simulink model "Copy_of_mVeh_fun_tbm"  (R2020a)
settings: configuration reference "config_10ms" (kept outside this file)
undefined symbols (not defined in the file): Calib_tbmVeh_drCmdMcP_incRate, Calib_tbmVeh_drCmdMcP_tgt, Calib_tbmVeh_set1_x4, Calib_tbmVeh_set2_x4, Parm_tbmVeh_sig_max_numInvalid, Parm_tbmVeh_sig_tolerate_numInvalid
libraries: canmsglib x7, speedgoatlib_IO691 x6, simulink x2, lib_signals_to_nByteLayout_withCrc x2, lib_cal_CAN_msgCount x2
settings Model: PauseTimes=49.73  NumberOfSteps=20  Creator=jianjun.gao  LastModifiedBy=bowen.zheng
settings ConfigSetRef: SourceName=config_10ms  SourceLocation=Base Workspace

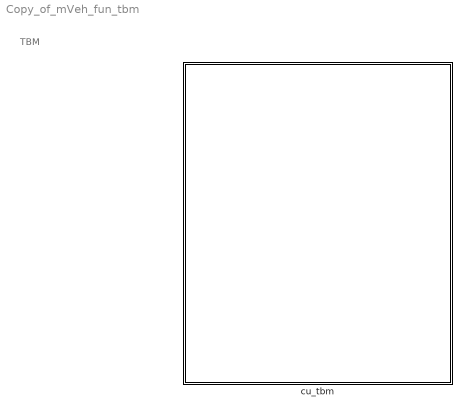
== system Copy_of_mVeh_fun_tbm ==
  note: TBM
  cu_tbm : Subsystem

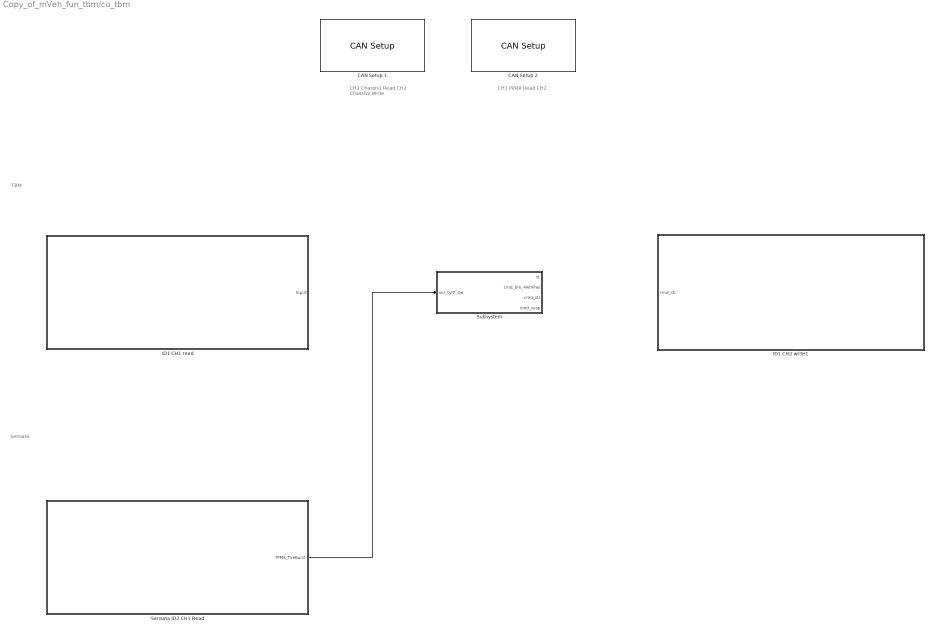
== system Copy_of_mVeh_fun_tbm/cu_tbm ==
  note: CH1 PVRR Read
      | CH2
  note: CH1 Chassis1 Read
      | CH2 Chassis2 Write
  note: Sensata
  note: TBM
  CAN Setup 1 : speedgoatlib_IO691/CAN Setup   moduletype=IO691  id=1  pciSlot=[12 0]  chn1=CAN (HS)  chn2=CAN (HS)  chn3=Disabled  chn4=Disabled  initStruct=[]  termStruct=[]  ArbitrationbdrChn1=500 kBaud  ArbitrationManbdrChn1=[2,16,63,16]  FdbdrChn1=5.0 MBaud  FdManbdrChn1=[2,2,5,2]  ArbitrationbdrChn2=500 kBaud  ArbitrationManbdrChn2=[2,16,63,16]  FdbdrChn2=5.0 MBaud  FdManbdrChn2=[2,2,5,2]  ArbitrationbdrChn3=1.0 MBaud  ArbitrationManbdrChn3=[2,8,31,8]  FdbdrChn3=5.0 MBaud  FdManbdrChn3=[2,2,5,2]  ArbitrationbdrChn4=1.0 MBaud  ArbitrationManbdrChn4=[2,8,31,8]  FdbdrChn4=5.0 MBaud  FdManbdrChn4=[2,2,5,2]  moduleInitValues=[691 1 12 0]
      settings: SourceProductName=Simulink Real-Time: Speedgoat I/O Blockset
  CAN Setup 2 : speedgoatlib_IO691/CAN Setup   moduletype=IO691  id=2  pciSlot=[7 0]  chn1=CAN (HS)  chn2=CAN (HS)  chn3=Disabled  chn4=Disabled  initStruct=[]  termStruct=[]  ArbitrationbdrChn1=500 kBaud  ArbitrationManbdrChn1=[2,16,63,16]  FdbdrChn1=5.0 MBaud  FdManbdrChn1=[2,2,5,2]  ArbitrationbdrChn2=500 kBaud  ArbitrationManbdrChn2=[2,16,63,16]  FdbdrChn2=5.0 MBaud  FdManbdrChn2=[2,2,5,2]  ArbitrationbdrChn3=1.0 MBaud  ArbitrationManbdrChn3=[2,8,31,8]  FdbdrChn3=5.0 MBaud  FdManbdrChn3=[2,2,5,2]  ArbitrationbdrChn4=1.0 MBaud  ArbitrationManbdrChn4=[2,8,31,8]  FdbdrChn4=5.0 MBaud  FdManbdrChn4=[2,2,5,2]  moduleInitValues=[691 2 7 0]
      settings: SourceProductName=Simulink Real-Time: Speedgoat I/O Blockset
  ID1 CH1 read : Subsystem
  ID1 CH2 write1 : Subsystem
  Sensata ID2 CH1 Read : Subsystem
  Subsystem : Subsystem
  wires:
  Sensata ID2 CH1 Read/1(TPMS_TireBurst) -> Subsystem/1(snr_tyrP_4w)

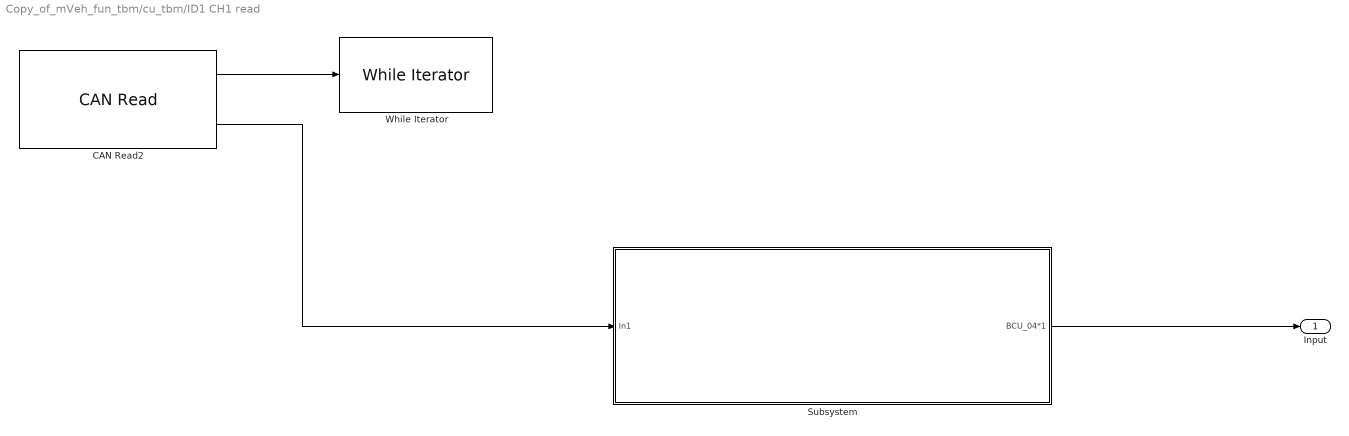
== system Copy_of_mVeh_fun_tbm/cu_tbm/ID1 CH1 read ==
  CAN Read2 : speedgoatlib_IO691/CAN Read  id=1  ts=-1  channel=1  messageType=CAN  canType=CAN (HS)  initValues=[691 1 -1 0 1 1]
      settings: SourceProductName=Simulink Real-Time: Speedgoat I/O Blockset
  Subsystem : Subsystem
  While Iterator : WhileIterator  MaxIters=-1  WhileBlockType=do-while
  Input : Outport
  wires:
  CAN Read2/1 -> While Iterator/1
  CAN Read2/2 -> Subsystem/1(In1)
  Subsystem/1(BCU_04*1) -> Input/1

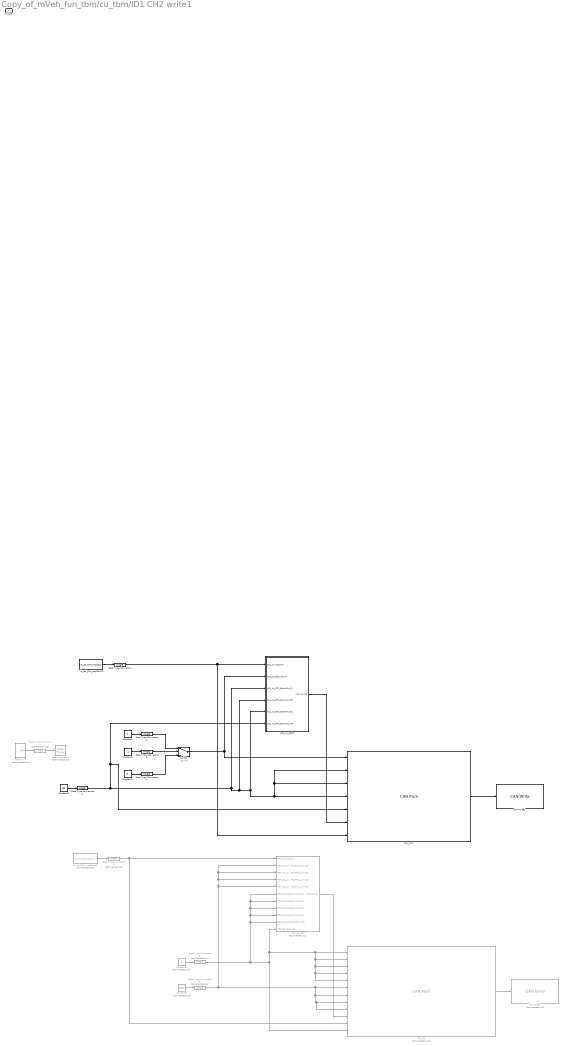
== system Copy_of_mVeh_fun_tbm/cu_tbm/ID1 CH2 write1 ==
  cmd_str : Inport
  CAN Write1 : speedgoatlib_IO691/CAN Write  id=1  ts=0.01  channel=2  messageType=CAN  enableStatusPort=off  canType=CAN (HS)  initValues=[691 1 0.01 1 1 1 0]
      settings: SourceProductName=Simulink Real-Time: Speedgoat I/O Blockset
  CAN Write2 : speedgoatlib_IO691/CAN Write  Commented=on  id=1  ts=0.01  channel=2  messageType=CAN  enableStatusPort=off  canType=CAN (HS)  initValues=[691 1 0.01 1 1 1 0]
      settings: SourceProductName=Simulink Real-Time: Speedgoat I/O Blockset
  Constant : Constant
  Constant1 : Constant  Value=0
  Constant2 : Constant  Value=80
  Constant3 : Constant  Commented=on  Value=2000
  Constant4 : Constant  Value=-1
  Constant6 : Constant  Commented=on
  Data Type Conversion{,2,4,7..8} (5 alike) : DataTypeConversion  OutDataTypeStr=single
  Data Type Conversion{1,3,5..6} (4 alike) : DataTypeConversion  Commented=on  OutDataTypeStr=single
  Gain (t) : Subsystem  Commented=on
  Rate Transition2 : RateTransition  Commented=on
  Switch : Switch  Criteria=u2 > Threshold
  TBM_02 : canmsglib/CAN Pack  Commented=on  CANdbFile=D:\spdGoat_prj_20221209\mVeh_fun_tbm_20221209\support\dbc\FCC1_NT2_Chassis1_CAN_Official_Release_V_1_4_DA_01_updated_mod.dbc  MsgList=TBM_02  MsgName=TBM_02  MsgIDType=Standard (11-bit identifier)  MsgIdentifier=128  MsgLength=8  Remote=off  ApplyMinMax=off  BusOutput=off  SignalInfo={'LeakActv_spring1','56','1','BE','unsigned','Standard','0','1','0','0','1';'LeakActv_spring2','57','1','BE','unsigned','Standard','0','1','0','0','1';'LeakActv_spring3','58','1','BE','unsigned','Standard','0','1','0','0','1';'LeakActv_spring4','59','1','BE','unsigned','Standard','0','1','0','0','1';'LeakFirst_springID','60','3','BE','unsigned','Standard','0','1','0','0','7';'LeakTargPres_spring1','17','11','BE','unsigned','Standard','0','1','0','0','2047';'LeakTargPres_spring2','38','11','BE','unsigned','Standard','0','1','0','0','2047';'LeakTargPres_spring3','43','11','BE','unsigned','Standard','0','1','0','0','2047';'LeakTargPres_spring4','48','11','BE','unsigned','Standard','0','1','0','0','2047';'TBM_02_CRC','0','8','BE','unsigned','Standard','0','1','0','0','255';'TBM_02_MsgCntr','12','4','BE','unsigned','Standard','0','1','0','0','15';'TBM_02_reserved','63','1','BE','unsigned','Standard','0','1','0','0','1'}
      settings: SourceProductBaseCode=ME,VN  DataFormat=CANdb specified signals
  TBM_02_CRC : Subsystem  Commented=on
  VCU_14*1 : canmsglib/CAN Pack  CANdbFile=D:\spdGoat_prj_20221209\mVeh_fun_tbm_20221209\support\dbc\NIO_NT2_Chassis2_CAN_Official_Release_V_1_1_DA_02.dbc  MsgList=VCU_14  MsgName=VCU_14  MsgIDType=Standard (11-bit identifier)  MsgIdentifier=75  MsgLength=8  Remote=off  ApplyMinMax=off  BusOutput=off  SignalInfo={'BTS_Active','23','1','BE','unsigned','Standard','0','1','0','0','1';'BTS_BrakeTar_FL','16','7','BE','unsigned','Standard','0','1','0','0','127';'BTS_BrakeTar_FR','25','7','BE','unsigned','Standard','0','1','0','0','127';'BTS_BrakeTar_RL','34','7','BE','unsigned','Standard','0','1','0','0','127';'BTS_BrakeTar_RR','43','7','BE','unsigned','Standard','0','1','0','0','127';'VCU_14_CRC','0','8','BE','unsigned','Standard','0','1','0','0','255';'VCU_14_MsgCntr','12','4','BE','unsigned','Standard','0','1','0','0','15'}
      settings: SourceProductBaseCode=ME,VN  DataFormat=CANdb specified signals
  VCU_14_CRC1 : Subsystem
  lib_cal_CAN_msgCount : lib_cal_CAN_msgCount/lib_cal_CAN_msgCount  SystemSampleTime=-1  Latency=0  AutoFrameSizeCalculation=off
  lib_cal_CAN_msgCount1 : lib_cal_CAN_msgCount/lib_cal_CAN_msgCount  Commented=on  SystemSampleTime=-1  Latency=0  AutoFrameSizeCalculation=off
  wires:
  Gain (t)/1("Gain ") -> Data Type Conversion1/1
  Constant/1 -> Data Type Conversion4/1
  Constant1/1 -> Data Type Conversion7/1
  Switch/1 -> VCU_14*1/1, VCU_14_CRC1/2("VCU_14_BTS_Active ")
  Constant2/1 -> Data Type Conversion2/1
  VCU_14_CRC1/1(VCU_14_crc) -> VCU_14*1/6
  Data Type Conversion/1 -> VCU_14*1/7, VCU_14_CRC1/1("VCU_14_MsgCntr ")
  lib_cal_CAN_msgCount/1 -> Data Type Conversion/1
  VCU_14*1/1 -> CAN Write1/1
  Data Type Conversion1/1 -> Rate Transition2/1
  Data Type Conversion2/1 -> VCU_14_CRC1/6("VCU_14_BTS_BrakeTar_RR "), VCU_14*1/5, VCU_14_CRC1/4("VCU_14_BTS_BrakeTar_FR "), VCU_14_CRC1/5("VCU_14_BTS_BrakeTar_RL "), VCU_14*1/2, VCU_14*1/3, VCU_14*1/4, VCU_14_CRC1/3("VCU_14_BTS_BrakeTar_FL ")
  TBM_02/1 -> CAN Write2/1
  Constant6/1 -> Data Type Conversion5/1
  TBM_02_CRC/1(TBM_02_crc) -> TBM_02/10
  lib_cal_CAN_msgCount1/1 -> Data Type Conversion3/1
  Constant3/1 -> Data Type Conversion6/1
  Data Type Conversion6/1 -> TBM_02_CRC/5("TBM_02_LeakTargPres_spring4 "), TBM_02_CRC/4("TBM_02_LeakTargPres_spring3 "), TBM_02_CRC/3("TBM_02_LeakTargPres_spring1 "), TBM_02_CRC/2("TBM_02_LeakTargPres_spring2 "), TBM_02/9, TBM_02/8, TBM_02/7, TBM_02/6
  Data Type Conversion3/1 -> TBM_02/11, TBM_02_CRC/1("TBM_02_MsgCntr ")
  Data Type Conversion5/1 -> TBM_02_CRC/10(TBM_02_LeakFirst_springID), TBM_02_CRC/9(TBM_02_LeakActv_spring3), TBM_02_CRC/8("TBM_02_LeakActv_spring4 "), TBM_02_CRC/6(TBM_02_LeakActv_spring2), TBM_02_CRC/7("TBM_02_LeakActv_spring1 "), TBM_02/12, TBM_02_CRC/11(TBM_02_reserved), TBM_02/5, TBM_02/4, TBM_02/3, TBM_02/2, TBM_02/1
  Data Type Conversion4/1 -> Switch/1
  Data Type Conversion7/1 -> Switch/3
  Constant4/1 -> Data Type Conversion8/1
  Data Type Conversion8/1 -> Switch/2

== system Copy_of_mVeh_fun_tbm/cu_tbm/Sensata ID2 CH1 Read ==
  CAN Read2 : speedgoatlib_IO691/CAN Read  id=2  ts=-1  channel=1  messageType=CAN  canType=CAN (HS)  initValues=[691 2 -1 0 1 1]
      settings: SourceProductName=Simulink Real-Time: Speedgoat I/O Blockset
  Subsystem : Subsystem
  While Iterator : WhileIterator  MaxIters=-1  WhileBlockType=do-while
  TPMS_TireBurst : Outport
  wires:
  CAN Read2/1 -> While Iterator/1
  CAN Read2/2 -> Subsystem/1(In1)
  Subsystem/1(TPMS_TireBurst) -> TPMS_TireBurst/1

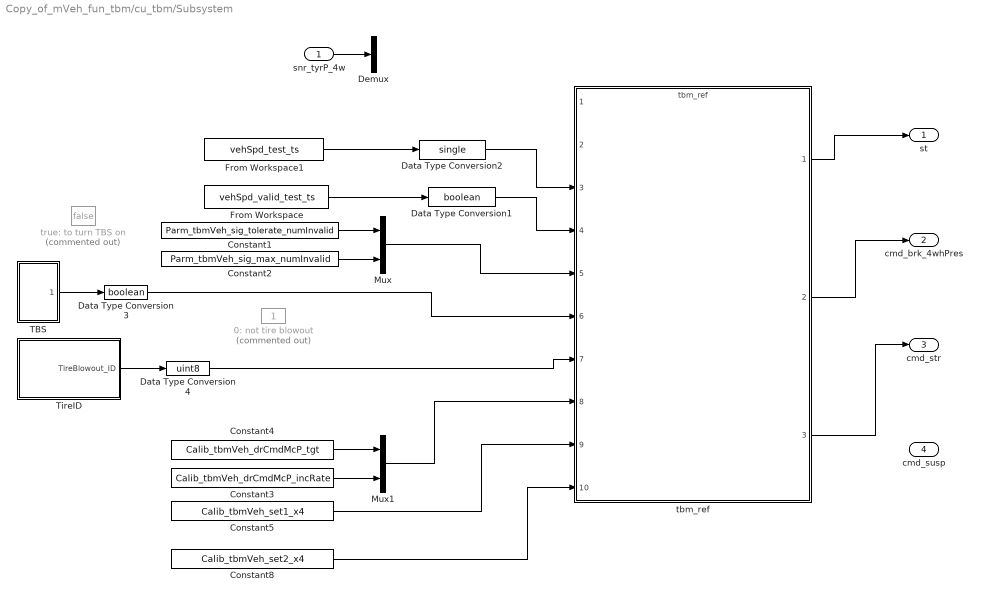
== system Copy_of_mVeh_fun_tbm/cu_tbm/Subsystem ==
  snr_tyrP_4w : Inport
  0: not tire blowout : Constant  Commented=on  OutDataTypeStr=uint8  SampleTime=-1
  Constant1 : Constant  Value=Parm_tbmVeh_sig_tolerate_numInvalid  OutDataTypeStr=int8  SampleTime=-1
  Constant2 : Constant  Value=Parm_tbmVeh_sig_max_numInvalid  OutDataTypeStr=int8  SampleTime=-1
  Constant3 : Constant  Value=Calib_tbmVeh_drCmdMcP_incRate  OutDataTypeStr=single  SampleTime=-1
  Constant4 : Constant  Value=Calib_tbmVeh_drCmdMcP_tgt  OutDataTypeStr=single  SampleTime=-1
  Constant5 : Constant  Value=Calib_tbmVeh_set1_x4  OutDataTypeStr=single  SampleTime=-1
  Constant8 : Constant  Value=Calib_tbmVeh_set2_x4  OutDataTypeStr=single  SampleTime=-1
  Data Type Conversion1 : DataTypeConversion  OutDataTypeStr=boolean
  Data Type Conversion2 : DataTypeConversion  OutDataTypeStr=single
  Data Type Conversion3 : DataTypeConversion  OutDataTypeStr=boolean
  Data Type Conversion4 : DataTypeConversion  OutDataTypeStr=uint8
  Demux : Demux  Outputs=2
  From Workspace : FromWorkspace  VariableName=vehSpd_valid_test_ts
  From Workspace1 : FromWorkspace  VariableName=vehSpd_test_ts
  Mux : Mux  Inputs=2
  Mux1 : Mux  Inputs=2
  TBS : Subsystem
  TireID : Subsystem
  tbm_ref : ModelReference  ModelNameDialog=tbm_ref.slx  SimulationMode=Normal  ModelReferenceVersion=1.657
  true: to turn TBS on : Constant  Commented=on  Value=false  OutDataTypeStr=boolean  SampleTime=-1
  st : Outport
  cmd_brk_4whPres : Outport  Port=2
  cmd_str : Outport  Port=3
  cmd_susp : Outport  Port=4
  wires:
  From Workspace1/1 -> Data Type Conversion2/1
  Constant8/1 -> tbm_ref/10
  Data Type Conversion1/1 -> tbm_ref/4
  Mux1/1 -> tbm_ref/8
  Data Type Conversion2/1 -> tbm_ref/3
  Constant1/1 -> Mux/1
  Mux/1 -> tbm_ref/5
  Constant2/1 -> Mux/2
  Data Type Conversion4/1 -> tbm_ref/7
  tbm_ref/3 -> cmd_str/1
  Constant3/1 -> Mux1/2
  Constant4/1 -> Mux1/1
  tbm_ref/1 -> st/1
  Constant5/1 -> tbm_ref/9
  From Workspace/1 -> Data Type Conversion1/1
  tbm_ref/2 -> cmd_brk_4whPres/1
  TBS/1("TBS_control ") -> Data Type Conversion3/1
  Data Type Conversion3/1 -> tbm_ref/6
  TireID/1("TireBlowout_ID ") -> Data Type Conversion4/1
  snr_tyrP_4w/1 -> Demux/1

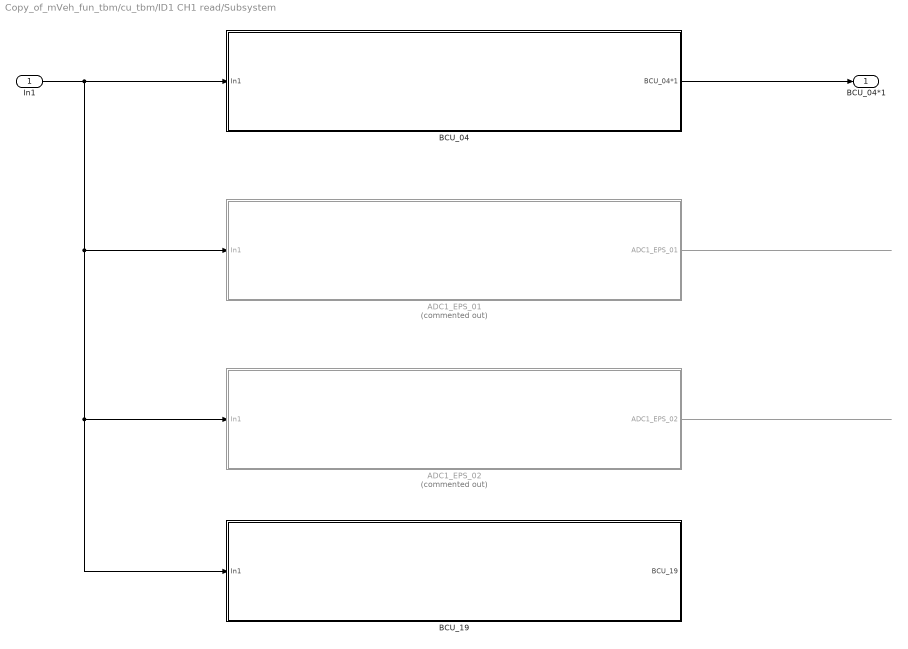
== system Copy_of_mVeh_fun_tbm/cu_tbm/ID1 CH1 read/Subsystem ==
  In1 : Inport
  ADC1_EPS_01 : Subsystem  Commented=on
  ADC1_EPS_02 : Subsystem  Commented=on
  BCU_04 : Subsystem
  BCU_19 : Subsystem
  BCU_04*1 : Outport
  wires:
  In1/1 -> BCU_19/1(In1), ADC1_EPS_02/1(In1), ADC1_EPS_01/1(In1), BCU_04/1(In1)
  ADC1_EPS_01/1(ADC1_EPS_01) -> ?
  ADC1_EPS_02/1(ADC1_EPS_02) -> ?
  BCU_04/1(BCU_04*1) -> BCU_04*1/1

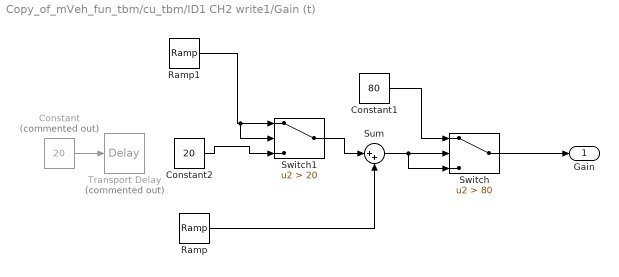
== system Copy_of_mVeh_fun_tbm/cu_tbm/ID1 CH2 write1/Gain (t) ==
  Constant : Constant  Commented=on  Value=20
  Constant1 : Constant  Value=80
  Constant2 : Constant  Value=20
  Ramp : simulink/Sources/Ramp  slope=60  start=20  InitialOutput=0
  Ramp1 : simulink/Sources/Ramp  slope=-600  start=10  InitialOutput=80
  Sum : Sum  Inputs=|++
  Switch : Switch  Criteria=u2 > Threshold  Threshold=80
  Switch1 : Switch  Criteria=u2 > Threshold  Threshold=20
  Transport Delay : TransportDelay  Commented=on  DelayTime=10  InitialOutput=80
  "Gain " : Outport
  wires:
  Constant1/1 -> Switch/1
  Ramp/1 -> Sum/2
  Sum/1 -> Switch/3, Switch/2
  Switch/1 -> "Gain "/1
  Constant/1 -> Transport Delay/1
  Ramp1/1 -> Switch1/2, Switch1/1
  Constant2/1 -> Switch1/3
  Switch1/1 -> Sum/1

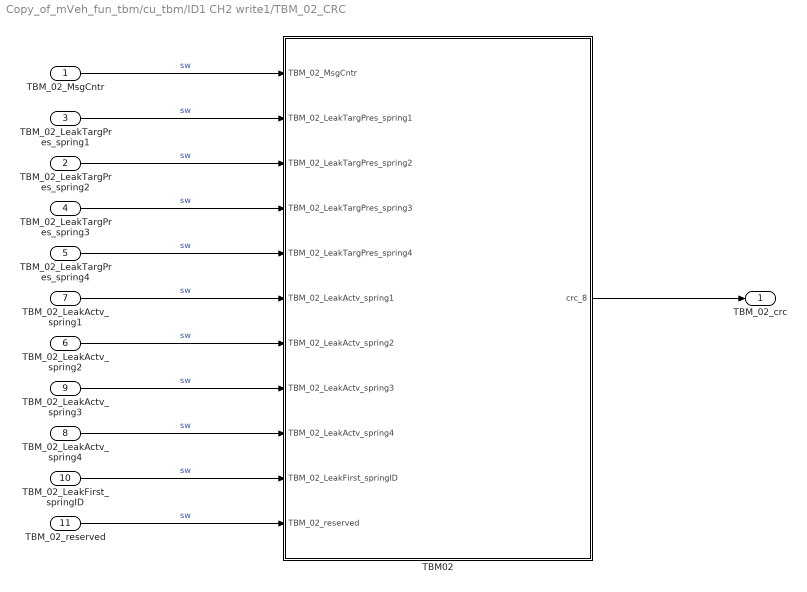
== system Copy_of_mVeh_fun_tbm/cu_tbm/ID1 CH2 write1/TBM_02_CRC ==
  "TBM_02_MsgCntr " : Inport
  "TBM_02_LeakTargPres_spring2 " : Inport  Port=2
  "TBM_02_LeakTargPres_spring1 " : Inport  Port=3
  "TBM_02_LeakTargPres_spring3 " : Inport  Port=4
  "TBM_02_LeakTargPres_spring4 " : Inport  Port=5
  TBM_02_LeakActv_spring2 : Inport  Port=6
  "TBM_02_LeakActv_spring1 " : Inport  Port=7
  "TBM_02_LeakActv_spring4 " : Inport  Port=8
  TBM_02_LeakActv_spring3 : Inport  Port=9
  TBM_02_LeakFirst_springID : Inport  Port=10
  TBM_02_reserved : Inport  Port=11
  TBM02 : Subsystem
  TBM_02_crc : Outport
  wires:
  "TBM_02_LeakTargPres_spring4 "/1 -> TBM02/5("TBM_02_LeakTargPres_spring4 ")  "sw"
  "TBM_02_LeakActv_spring1 "/1 -> TBM02/6("TBM_02_LeakActv_spring1 ")  "sw"
  "TBM_02_MsgCntr "/1 -> TBM02/1("TBM_02_MsgCntr ")  "sw"
  "TBM_02_LeakTargPres_spring1 "/1 -> TBM02/2("TBM_02_LeakTargPres_spring1 ")  "sw"
  "TBM_02_LeakTargPres_spring2 "/1 -> TBM02/3("TBM_02_LeakTargPres_spring2 ")  "sw"
  "TBM_02_LeakTargPres_spring3 "/1 -> TBM02/4("TBM_02_LeakTargPres_spring3 ")  "sw"
  TBM02/1(crc_8) -> TBM_02_crc/1
  "TBM_02_LeakActv_spring4 "/1 -> TBM02/9("TBM_02_LeakActv_spring4 ")  "sw"
  TBM_02_LeakActv_spring3/1 -> TBM02/8("TBM_02_LeakActv_spring3 ")  "sw"
  TBM_02_LeakActv_spring2/1 -> TBM02/7(TBM_02_LeakActv_spring2)  "sw"
  TBM_02_reserved/1 -> TBM02/11("TBM_02_reserved ")  "sw"
  TBM_02_LeakFirst_springID/1 -> TBM02/10(TBM_02_LeakFirst_springID)  "sw"

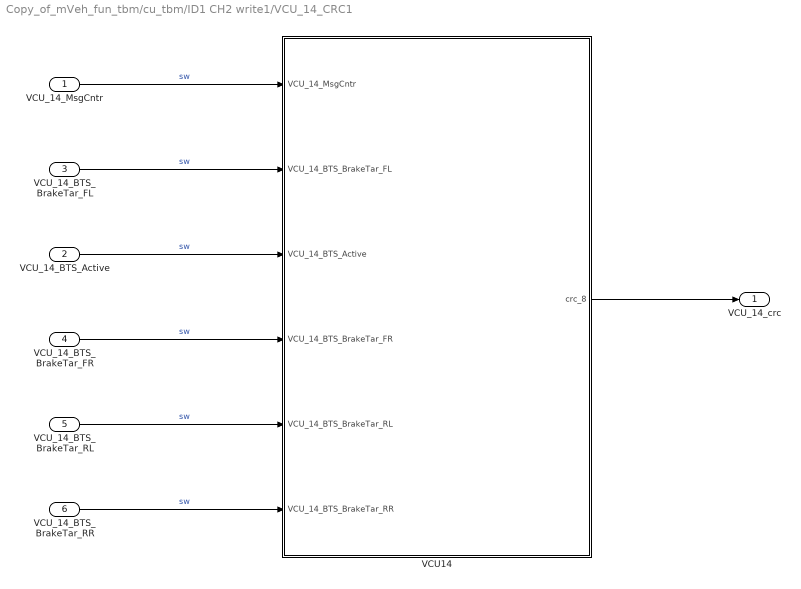
== system Copy_of_mVeh_fun_tbm/cu_tbm/ID1 CH2 write1/VCU_14_CRC1 ==
  "VCU_14_MsgCntr " : Inport
  "VCU_14_BTS_Active " : Inport  Port=2
  "VCU_14_BTS_BrakeTar_FL " : Inport  Port=3
  "VCU_14_BTS_BrakeTar_FR " : Inport  Port=4
  "VCU_14_BTS_BrakeTar_RL " : Inport  Port=5
  "VCU_14_BTS_BrakeTar_RR " : Inport  Port=6
  VCU14 : Subsystem
  VCU_14_crc : Outport
  wires:
  "VCU_14_BTS_BrakeTar_RL "/1 -> VCU14/5("VCU_14_BTS_BrakeTar_RL ")  "sw"
  "VCU_14_BTS_BrakeTar_RR "/1 -> VCU14/6("VCU_14_BTS_BrakeTar_RR ")  "sw"
  "VCU_14_MsgCntr "/1 -> VCU14/1("VCU_14_MsgCntr ")  "sw"
  "VCU_14_BTS_BrakeTar_FL "/1 -> VCU14/2("VCU_14_BTS_BrakeTar_FL ")  "sw"
  "VCU_14_BTS_Active "/1 -> VCU14/3("VCU_14_BTS_Active ")  "sw"
  "VCU_14_BTS_BrakeTar_FR "/1 -> VCU14/4("VCU_14_BTS_BrakeTar_FR ")  "sw"
  VCU14/1(crc_8) -> VCU_14_crc/1

== system Copy_of_mVeh_fun_tbm/cu_tbm/Sensata ID2 CH1 Read/Subsystem ==
  In1 : Inport
  TPMS_TireBurst_Matrix : Subsystem
  TPMS_TireBurst : Outport
  wires:
  In1/1 -> TPMS_TireBurst_Matrix/1(In1)
  TPMS_TireBurst_Matrix/1(TPMS_TireBurst*1) -> TPMS_TireBurst/1

== system Copy_of_mVeh_fun_tbm/cu_tbm/Subsystem/TBS ==
  Constant2 : Constant
  Transport Delay : TransportDelay
  "TBS_control " : Outport
  wires:
  Constant2/1 -> Transport Delay/1
  Transport Delay/1 -> "TBS_control "/1

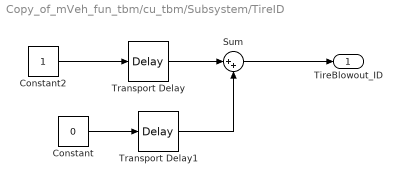
== system Copy_of_mVeh_fun_tbm/cu_tbm/Subsystem/TireID ==
  Constant : Constant  Value=0
  Constant2 : Constant
  Sum : Sum  Inputs=|++
  Transport Delay : TransportDelay  DelayTime=2
  Transport Delay1 : TransportDelay  DelayTime=11
  "TireBlowout_ID " : Outport
  wires:
  Constant2/1 -> Transport Delay/1
  Transport Delay/1 -> Sum/1
  Sum/1 -> "TireBlowout_ID "/1
  Constant/1 -> Transport Delay1/1
  Transport Delay1/1 -> Sum/2

== system Copy_of_mVeh_fun_tbm/cu_tbm/ID1 CH1 read/Subsystem/ADC1_EPS_01 ==
  In1 : Inport
  Bus Creator : BusCreator  Inputs=11
  Chassis 1 ADC1_EPS_01 : canmsglib/CAN Unpack  CANdbFile=D:\spdGoat_prj_20221103\NIO_NT2_Chassis1_CAN_Official_Release_V_1_1_DA_02.dbc  MsgList=ADC1_EPS_01  MsgName=ADC1_EPS_01  MsgIDType=Standard (11-bit identifier)  MsgIdentifier=112  MsgLength=8  SignalInfo={'ADC1_EPSACIRampRate','57','2','BE','unsigned','Standard','0','1','0','0','3';'ADC1_EPSACIReq','41','15','BE','unsigned','Standard','0','0.1','-1638.4','-1638.4','1638.3';'ADC1_EPSACIReqVal','40','1','BE','unsigned','Standard','0','1','0','0','1';'ADC1_EPSACISafLim_AngDyn','25','15','BE','unsigned','Standard','0','0.1','-1638.4','-1638.4','1638.3';'ADC1_EPSACISafLim_AngDynOffs','8','4','BE','unsigned','Standard','0','1','0','0','15';'ADC1_EPSACISafLim_AngLM','52','4','BE','unsigned','Standard','0','1','0','0','15';'ADC1_EPSACISafLim_AngRM','48','4','BE','unsigned','Standard','0','1','0','0','15';'ADC1_EPSACISafLim_Mode','24','1','BE','unsigned','Standard','0','1','0','0','1';'ADC1_EPSACISafLim_Rate','59','5','BE','unsigned','Standard','0','1','0','0','31';'ADC1_EPS_01_CRC','0','8','BE','unsigned','Standard','0','1','0','0','255';'ADC1_EPS_01_MsgCntr','12','4','BE','unsigned','Standard','0','1','0','0','15'}  IDPort=off  TimestampPort=off  ErrorPort=off  RemotePort=off  LengthPort=off  StatusPort=off  ApplyMinMax=off
      settings: SourceProductBaseCode=ME,VN  DataFormat=CANdb specified signals
  ADC1_EPS_01 : Outport
  wires:
  Bus Creator/1 -> ADC1_EPS_01/1  "ADC1_EPS_01"
  In1/1 -> Chassis 1 ADC1_EPS_01/1
  Chassis 1 ADC1_EPS_01/10 -> Bus Creator/10  "EPS_01_CRC"
  Chassis 1 ADC1_EPS_01/3 -> Bus Creator/3  "EPSACIReqVal"
  Chassis 1 ADC1_EPS_01/9 -> Bus Creator/9  "EPSACISafLim_Rate"
  Chassis 1 ADC1_EPS_01/4 -> Bus Creator/4  "EPSACISafLim_AngDyn"
  Chassis 1 ADC1_EPS_01/1 -> Bus Creator/1  "EPSACIRampRate"
  Chassis 1 ADC1_EPS_01/5 -> Bus Creator/5  "EPSACISafLim_AngDynOffs"
  Chassis 1 ADC1_EPS_01/7 -> Bus Creator/7  "EPSACISafLim_AngRM"
  Chassis 1 ADC1_EPS_01/11 -> Bus Creator/11  "EPS_01_MsgCntr"
  Chassis 1 ADC1_EPS_01/2 -> Bus Creator/2  "EPSACIReq"
  Chassis 1 ADC1_EPS_01/8 -> Bus Creator/8  "EPSACISafLim_Mode"
  Chassis 1 ADC1_EPS_01/6 -> Bus Creator/6  "EPSACISafLim_AngLM"

== system Copy_of_mVeh_fun_tbm/cu_tbm/ID1 CH1 read/Subsystem/ADC1_EPS_02 ==
  In1 : Inport
  Bus Creator : BusCreator  Inputs=9
  Chassis 1 ADC1_EPS_02 : canmsglib/CAN Unpack  CANdbFile=D:\spdGoat_prj_20221103\NIO_NT2_Chassis1_CAN_Official_Release_V_1_1_DA_02.dbc  MsgList=ADC1_EPS_02  MsgName=ADC1_EPS_02  MsgIDType=Standard (11-bit identifier)  MsgIdentifier=113  MsgLength=8  SignalInfo={'ADC1_EPSACIOvrThr','18','3','BE','unsigned','Standard','0','1','0','0','7';'ADC1_EPSACITsuSup','21','3','BE','unsigned','Standard','0','1','0','0','7';'ADC1_EPSCTIReq','24','10','BE','unsigned','Standard','0','0.02','-10.24','-10.24','10.22';'ADC1_EPSCTIReqVal','39','1','BE','unsigned','Standard','0','1','0','0','1';'ADC1_EPSHVIReq','9','3','BE','unsigned','Standard','0','1','0','0','7';'ADC1_EPSHVIReqVal','8','1','BE','unsigned','Standard','0','1','0','0','1';'ADC1_EPSReqTyp','36','3','BE','unsigned','Standard','0','1','0','0','7';'ADC1_EPS_02_CRC','0','8','BE','unsigned','Standard','0','1','0','0','255';'ADC1_EPS_02_MsgCntr','12','4','BE','unsigned','Standard','0','1','0','0','15'}  IDPort=off  TimestampPort=off  ErrorPort=off  RemotePort=off  LengthPort=off  StatusPort=off  ApplyMinMax=off
      settings: SourceProductBaseCode=ME,VN  DataFormat=CANdb specified signals
  ADC1_EPS_02 : Outport
  wires:
  Bus Creator/1 -> ADC1_EPS_02/1  "ADC1_EPS_02"
  In1/1 -> Chassis 1 ADC1_EPS_02/1
  Chassis 1 ADC1_EPS_02/2 -> Bus Creator/2  "EPSACITsuSup"
  Chassis 1 ADC1_EPS_02/4 -> Bus Creator/4  "EPSCTIReqVal"
  Chassis 1 ADC1_EPS_02/3 -> Bus Creator/3  "EPSCTIReq"
  Chassis 1 ADC1_EPS_02/9 -> Bus Creator/9  "EPS_02_MsgCntr"
  Chassis 1 ADC1_EPS_02/8 -> Bus Creator/8  "EPS_02_CRC"
  Chassis 1 ADC1_EPS_02/5 -> Bus Creator/5  "EPSHVIReq"
  Chassis 1 ADC1_EPS_02/6 -> Bus Creator/6  "EPSHVIReqVal"
  Chassis 1 ADC1_EPS_02/1 -> Bus Creator/1  "EPSACIOvrThr"
  Chassis 1 ADC1_EPS_02/7 -> Bus Creator/7  "EPSReqTyp"

== system Copy_of_mVeh_fun_tbm/cu_tbm/ID1 CH1 read/Subsystem/BCU_04 ==
  In1 : Inport
  Bus Creator : BusCreator  Inputs=18
  Chassis 1 BCU_04 : canmsglib/CAN Unpack  CANdbFile=D:\spdGoat_prj_20221209\mVeh_fun_tbm_20221209\support\dbc\NIO_NT2_Chassis1_CAN_Official_Release_V_1_1_DA_02.dbc  MsgList=BCU_04  MsgName=BCU_04  MsgIDType=Standard (11-bit identifier)  MsgIdentifier=91  MsgLength=8  SignalInfo={'BCUBrkLiReq','9','2','BE','unsigned','Standard','0','1','0','0','3';'BCU_04_CRC','0','8','BE','unsigned','Standard','0','1','0','0','255';'BCU_04_MsgCntr','12','4','BE','unsigned','Standard','0','1','0','0','15';'BCU_NoBrkF','8','1','BE','unsigned','Standard','0','1','0','0','1';'BCU_SupInfo','48','2','BE','unsigned','Standard','0','1','0','0','3';'BrkOverHeat','50','1','BE','unsigned','Standard','0','1','0','0','1';'BrkPedlSts','54','2','BE','unsigned','Standard','0','1','0','0','3';'BrkPedlTrvl','56','8','BE','unsigned','Standard','0','0.4','0','0','102';'BrkPedlTrvlCalSts','52','2','BE','unsigned','Standard','0','1','0','0','3';'BrkPress','47','9','BE','unsigned','Standard','0','1','-42.5','-42.5','425.5';'BrkPressOffset','42','5','BE','unsigned','Standard','0','1','-15','-15','15';'BrkPressOffsetValid','41','1','BE','unsigned','Standard','0','1','0','0','1';'BrkPressValid','40','1','BE','unsigned','Standard','0','1','0','0','1';'HAZReq','11','1','BE','unsigned','Standard','0','1','0','0','1';'IPB_TwoFoot_DriveWarning','51','1','BE','unsigned','Standard','0','1','0','0','1';'VehMovgDir','21','2','BE','unsigned','Standard','0','1','0','0','3';'VehSpd','24','13','BE','unsigned','Standard','0','0.05625','0','0','360';'VehSpdSts','23','1','BE','unsigned','Standard','0','1','0','0','1'}  IDPort=off  TimestampPort=off  ErrorPort=off  RemotePort=off  LengthPort=off  StatusPort=off  ApplyMinMax=off
      settings: SourceProductBaseCode=ME,VN  DataFormat=CANdb specified signals
  BCU_04*1 : Outport
  wires:
  Chassis 1 BCU_04/8 -> Bus Creator/8  "BrkPedlTrvl"
  Chassis 1 BCU_04/3 -> Bus Creator/3  "BCU_04_MsgCntr"
  Chassis 1 BCU_04/2 -> Bus Creator/2  "BCU_04_CRC"
  Chassis 1 BCU_04/4 -> Bus Creator/4  "BCU_NoBrkF"
  Chassis 1 BCU_04/16 -> Bus Creator/16  "VehMovgDir"
  Chassis 1 BCU_04/11 -> Bus Creator/11  "BrkPressOffset"
  Chassis 1 BCU_04/7 -> Bus Creator/7  "BrkPedlSts"
  Chassis 1 BCU_04/13 -> Bus Creator/13  "BrkPressValid"
  Chassis 1 BCU_04/10 -> Bus Creator/10  "BrkPress"
  Chassis 1 BCU_04/6 -> Bus Creator/6  "BrkOverHeat"
  Chassis 1 BCU_04/5 -> Bus Creator/5  "BCU_SupInfo"
  Bus Creator/1 -> BCU_04*1/1  "BCU_04"
  Chassis 1 BCU_04/17 -> Bus Creator/17  "VehSpd"
  Chassis 1 BCU_04/14 -> Bus Creator/14  "HAZReq"
  Chassis 1 BCU_04/18 -> Bus Creator/18  "VehSpdSts"
  Chassis 1 BCU_04/1 -> Bus Creator/1  "BCUBrkLiReq"
  Chassis 1 BCU_04/9 -> Bus Creator/9  "BrkPedlTrvlCalSts"
  Chassis 1 BCU_04/15 -> Bus Creator/15  "IPB_TwoFoot_DriveWarning"
  Chassis 1 BCU_04/12 -> Bus Creator/12  "BrkPressOffsetValid"
  In1/1 -> Chassis 1 BCU_04/1

== system Copy_of_mVeh_fun_tbm/cu_tbm/ID1 CH1 read/Subsystem/BCU_19 ==
  In1 : Inport
  Bus Creator : BusCreator  Inputs=9
  Chassis 1 BCU_19 : canmsglib/CAN Unpack  CANdbFile=D:\spdGoat_prj_20221209\mVeh_fun_tbm_20221209\support\dbc\NIO_NT2_Chassis1_CAN_Official_Release_V_1_1_DA_02.dbc  MsgList=BCU_19  MsgName=BCU_19  MsgIDType=Standard (11-bit identifier)  MsgIdentifier=107  MsgLength=8  SignalInfo={'PSP_Pressure','56','12','BE','unsigned','Standard','0','0.05','-5','-5','199.75';'WheelBrkPFrntLe','12','12','BE','unsigned','Standard','0','0.1','0','0','409.5';'WheelBrkPFrntRi','16','12','BE','unsigned','Standard','0','0.1','0','0','409.5';'WheelBrkPReLe','36','12','BE','unsigned','Standard','0','0.1','0','0','409.5';'WheelBrkPReRi','40','12','BE','unsigned','Standard','0','0.1','0','0','409.5';'WheelBrkPReliabilityFrntLe','55','1','BE','unsigned','Standard','0','1','0','0','1';'WheelBrkPReliabilityFrntRi','54','1','BE','unsigned','Standard','0','1','0','0','1';'WheelBrkPReliabilityReLe','53','1','BE','unsigned','Standard','0','1','0','0','1';'WheelBrkPReliabilityReRi','52','1','BE','unsigned','Standard','0','1','0','0','1'}  IDPort=off  TimestampPort=off  ErrorPort=off  RemotePort=off  LengthPort=off  StatusPort=off  ApplyMinMax=off
      settings: SourceProductBaseCode=ME,VN  DataFormat=CANdb specified signals
  BCU_19 : Outport
  wires:
  Chassis 1 BCU_19/8 -> Bus Creator/8  "WheelBrkPReliabilityReLe"
  Chassis 1 BCU_19/3 -> Bus Creator/3  "WheelBrkPFrntRi"
  Chassis 1 BCU_19/2 -> Bus Creator/2  "WheelBrkPFrntLe"
  Chassis 1 BCU_19/4 -> Bus Creator/4  "WheelBrkPReLe"
  Chassis 1 BCU_19/7 -> Bus Creator/7  "WheelBrkPReliabilityFrntRi"
  Chassis 1 BCU_19/6 -> Bus Creator/6  "WheelBrkPReliabilityFrntLe"
  Chassis 1 BCU_19/5 -> Bus Creator/5  "WheelBrkPReRi"
  Bus Creator/1 -> BCU_19/1  "BCU_19"
  Chassis 1 BCU_19/1 -> Bus Creator/1  "PSP_Pressure"
  Chassis 1 BCU_19/9 -> Bus Creator/9  "WheelBrkPReliabilityReRi"
  In1/1 -> Chassis 1 BCU_19/1

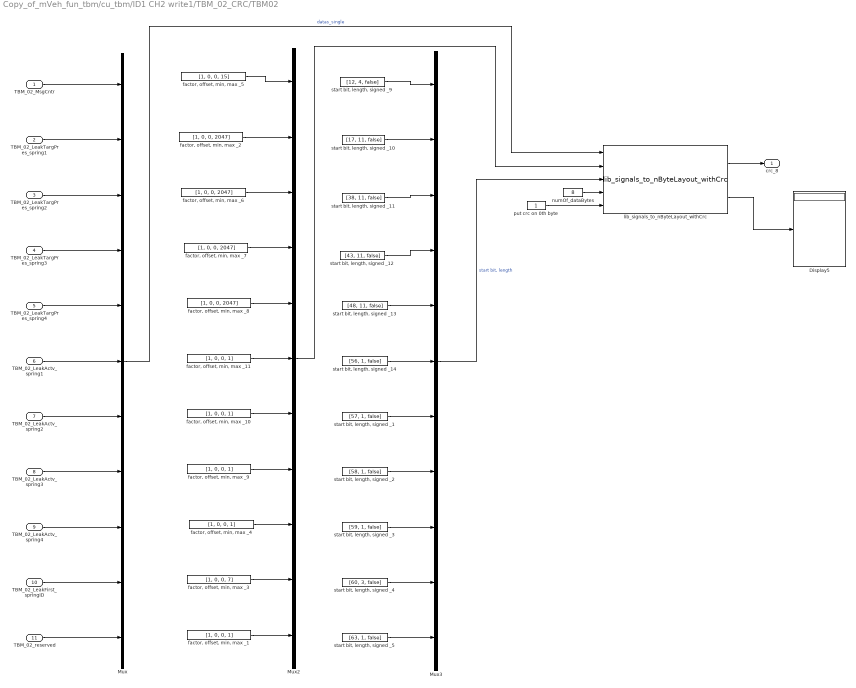
== system Copy_of_mVeh_fun_tbm/cu_tbm/ID1 CH2 write1/TBM_02_CRC/TBM02 ==
  "TBM_02_MsgCntr " : Inport
  "TBM_02_LeakTargPres_spring1 " : Inport  Port=2
  "TBM_02_LeakTargPres_spring2 " : Inport  Port=3
  "TBM_02_LeakTargPres_spring3 " : Inport  Port=4
  "TBM_02_LeakTargPres_spring4 " : Inport  Port=5
  "TBM_02_LeakActv_spring1 " : Inport  Port=6
  TBM_02_LeakActv_spring2 : Inport  Port=7
  "TBM_02_LeakActv_spring3 " : Inport  Port=8
  "TBM_02_LeakActv_spring4 " : Inport  Port=9
  TBM_02_LeakFirst_springID : Inport  Port=10
  "TBM_02_reserved " : Inport  Port=11
  Display5 : Display
  Mux : Mux  Inputs=11
  Mux2 : Mux  Inputs=11
  Mux3 : Mux  Inputs=11
  factor, offset, min, max _{1,4,9..11} (5 alike) : Constant  Value=[1, 0, 0, 1]  OutDataTypeStr=single  SampleTime=-1
  factor, offset, min, max _{2,6..8} (4 alike) : Constant  Value=[1, 0, 0, 2047]  OutDataTypeStr=single  SampleTime=-1
  "factor, offset, min, max _3" : Constant  Value=[1, 0, 0, 7]  OutDataTypeStr=single  SampleTime=-1
  "factor, offset, min, max _5" : Constant  Value=[1, 0, 0, 15]  OutDataTypeStr=single  SampleTime=-1
  lib_signals_to_nByteLayout_withCrc : lib_signals_to_nByteLayout_withCrc/lib_signals_to_nByteLayout_withCrc  SystemSampleTime=-1  Latency=0  AutoFrameSizeCalculation=off
  numOf_dataBytes : Constant  Value=8  OutDataTypeStr=uint8  SampleTime=-1
  put crc on 0th byte : Constant  OutDataTypeStr=uint8  SampleTime=-1
  "start bit, length, signed _1" : Constant  Value=[57, 1, false]  OutDataTypeStr=uint8  SampleTime=-1
  "start bit, length, signed _10" : Constant  Value=[17, 11, false]  OutDataTypeStr=uint8  SampleTime=-1
  "start bit, length, signed _11" : Constant  Value=[38, 11, false]  OutDataTypeStr=uint8  SampleTime=-1
  "start bit, length, signed _12" : Constant  Value=[43, 11, false]  OutDataTypeStr=uint8  SampleTime=-1
  "start bit, length, signed _13" : Constant  Value=[48, 11, false]  OutDataTypeStr=uint8  SampleTime=-1
  "start bit, length, signed _14" : Constant  Value=[56, 1, false]  OutDataTypeStr=uint8  SampleTime=-1
  "start bit, length, signed _2" : Constant  Value=[58, 1, false]  OutDataTypeStr=uint8  SampleTime=-1
  "start bit, length, signed _3" : Constant  Value=[59, 1, false]  OutDataTypeStr=uint8  SampleTime=-1
  "start bit, length, signed _4" : Constant  Value=[60, 3, false]  OutDataTypeStr=uint8  SampleTime=-1
  "start bit, length, signed _5" : Constant  Value=[63, 1, false]  OutDataTypeStr=uint8  SampleTime=-1
  "start bit, length, signed _9" : Constant  Value=[12, 4, false]  OutDataTypeStr=uint8  SampleTime=-1
  crc_8 : Outport
  wires:
  "TBM_02_LeakTargPres_spring1 "/1 -> Mux/2
  "TBM_02_LeakTargPres_spring4 "/1 -> Mux/5
  "start bit, length, signed _12"/1 -> Mux3/4
  Mux/1 -> lib_signals_to_nByteLayout_withCrc/1  "datas_single"
  "start bit, length, signed _13"/1 -> Mux3/5
  "TBM_02_MsgCntr "/1 -> Mux/1
  "TBM_02_LeakTargPres_spring3 "/1 -> Mux/4
  "start bit, length, signed _11"/1 -> Mux3/3
  "start bit, length, signed _9"/1 -> Mux3/1
  lib_signals_to_nByteLayout_withCrc/2 -> Display5/1
  "start bit, length, signed _14"/1 -> Mux3/6
  "TBM_02_LeakTargPres_spring2 "/1 -> Mux/3
  Mux3/1 -> lib_signals_to_nByteLayout_withCrc/3  "start bit, length"
  "factor, offset, min, max _2"/1 -> Mux2/2
  put crc on 0th byte/1 -> lib_signals_to_nByteLayout_withCrc/5
  "factor, offset, min, max _6"/1 -> Mux2/3
  "factor, offset, min, max _5"/1 -> Mux2/1
  Mux2/1 -> lib_signals_to_nByteLayout_withCrc/2
  "start bit, length, signed _10"/1 -> Mux3/2
  "TBM_02_LeakActv_spring1 "/1 -> Mux/6
  lib_signals_to_nByteLayout_withCrc/1 -> crc_8/1
  numOf_dataBytes/1 -> lib_signals_to_nByteLayout_withCrc/4
  "factor, offset, min, max _7"/1 -> Mux2/4
  "factor, offset, min, max _8"/1 -> Mux2/5
  "factor, offset, min, max _11"/1 -> Mux2/6
  TBM_02_LeakActv_spring2/1 -> Mux/7
  "TBM_02_LeakActv_spring3 "/1 -> Mux/8
  TBM_02_LeakFirst_springID/1 -> Mux/10
  "TBM_02_reserved "/1 -> Mux/11
  "TBM_02_LeakActv_spring4 "/1 -> Mux/9
  "factor, offset, min, max _1"/1 -> Mux2/11
  "factor, offset, min, max _3"/1 -> Mux2/10
  "factor, offset, min, max _4"/1 -> Mux2/9
  "factor, offset, min, max _9"/1 -> Mux2/8
  "factor, offset, min, max _10"/1 -> Mux2/7
  "start bit, length, signed _1"/1 -> Mux3/7
  "start bit, length, signed _2"/1 -> Mux3/8
  "start bit, length, signed _3"/1 -> Mux3/9
  "start bit, length, signed _4"/1 -> Mux3/10
  "start bit, length, signed _5"/1 -> Mux3/11

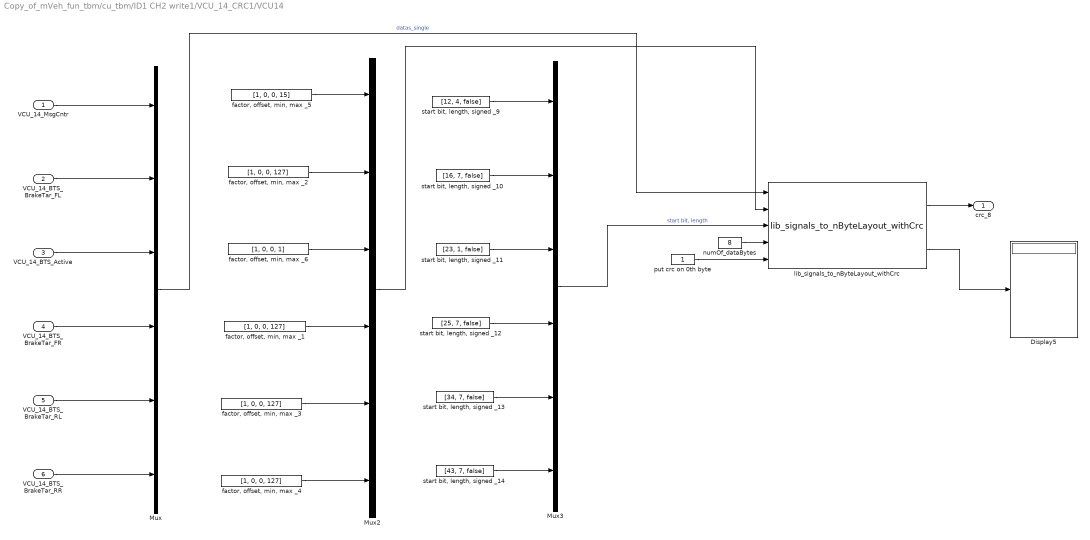
== system Copy_of_mVeh_fun_tbm/cu_tbm/ID1 CH2 write1/VCU_14_CRC1/VCU14 ==
  "VCU_14_MsgCntr " : Inport
  "VCU_14_BTS_BrakeTar_FL " : Inport  Port=2
  "VCU_14_BTS_Active " : Inport  Port=3
  "VCU_14_BTS_BrakeTar_FR " : Inport  Port=4
  "VCU_14_BTS_BrakeTar_RL " : Inport  Port=5
  "VCU_14_BTS_BrakeTar_RR " : Inport  Port=6
  Display5 : Display
  Mux : Mux  Inputs=6
  Mux2 : Mux  Inputs=6
  Mux3 : Mux  Inputs=6
  factor, offset, min, max _{1..4} (4 alike) : Constant  Value=[1, 0, 0, 127]  OutDataTypeStr=single  SampleTime=-1
  "factor, offset, min, max _5" : Constant  Value=[1, 0, 0, 15]  OutDataTypeStr=single  SampleTime=-1
  "factor, offset, min, max _6" : Constant  Value=[1, 0, 0, 1]  OutDataTypeStr=single  SampleTime=-1
  lib_signals_to_nByteLayout_withCrc : lib_signals_to_nByteLayout_withCrc/lib_signals_to_nByteLayout_withCrc  SystemSampleTime=-1  Latency=0  AutoFrameSizeCalculation=off
  numOf_dataBytes : Constant  Value=8  OutDataTypeStr=uint8  SampleTime=-1
  put crc on 0th byte : Constant  OutDataTypeStr=uint8  SampleTime=-1
  "start bit, length, signed _10" : Constant  Value=[16, 7, false]  OutDataTypeStr=uint8  SampleTime=-1
  "start bit, length, signed _11" : Constant  Value=[23, 1, false]  OutDataTypeStr=uint8  SampleTime=-1
  "start bit, length, signed _12" : Constant  Value=[25, 7, false]  OutDataTypeStr=uint8  SampleTime=-1
  "start bit, length, signed _13" : Constant  Value=[34, 7, false]  OutDataTypeStr=uint8  SampleTime=-1
  "start bit, length, signed _14" : Constant  Value=[43, 7, false]  OutDataTypeStr=uint8  SampleTime=-1
  "start bit, length, signed _9" : Constant  Value=[12, 4, false]  OutDataTypeStr=uint8  SampleTime=-1
  crc_8 : Outport
  wires:
  "VCU_14_BTS_BrakeTar_FL "/1 -> Mux/2
  "VCU_14_BTS_BrakeTar_RL "/1 -> Mux/5
  "start bit, length, signed _12"/1 -> Mux3/4
  Mux/1 -> lib_signals_to_nByteLayout_withCrc/1  "datas_single"
  "start bit, length, signed _13"/1 -> Mux3/5
  "VCU_14_MsgCntr "/1 -> Mux/1
  "VCU_14_BTS_BrakeTar_FR "/1 -> Mux/4
  "start bit, length, signed _11"/1 -> Mux3/3
  "start bit, length, signed _9"/1 -> Mux3/1
  lib_signals_to_nByteLayout_withCrc/2 -> Display5/1
  "start bit, length, signed _14"/1 -> Mux3/6
  "VCU_14_BTS_Active "/1 -> Mux/3
  Mux3/1 -> lib_signals_to_nByteLayout_withCrc/3  "start bit, length"
  "factor, offset, min, max _2"/1 -> Mux2/2
  put crc on 0th byte/1 -> lib_signals_to_nByteLayout_withCrc/5
  "factor, offset, min, max _6"/1 -> Mux2/3
  "factor, offset, min, max _5"/1 -> Mux2/1
  Mux2/1 -> lib_signals_to_nByteLayout_withCrc/2
  "start bit, length, signed _10"/1 -> Mux3/2
  "VCU_14_BTS_BrakeTar_RR "/1 -> Mux/6
  lib_signals_to_nByteLayout_withCrc/1 -> crc_8/1
  numOf_dataBytes/1 -> lib_signals_to_nByteLayout_withCrc/4
  "factor, offset, min, max _1"/1 -> Mux2/4
  "factor, offset, min, max _3"/1 -> Mux2/5
  "factor, offset, min, max _4"/1 -> Mux2/6

== system Copy_of_mVeh_fun_tbm/cu_tbm/Sensata ID2 CH1 Read/Subsystem/TPMS_TireBurst_Matrix ==
  In1 : Inport
  Bus Creator : BusCreator  Inputs=8
  TPMS_TireBurst : canmsglib/CAN Unpack  CANdbFile=D:\spdGoat_prj_20221215\mVeh_fun_tbm_20221215\support\dbc\NIO_TPMS_TireBurst_Matrix_V1.0.dbc  MsgList=TMPS_TireBurst_Msg  MsgName=TMPS_TireBurst_Msg  MsgIDType=Standard (11-bit identifier)  MsgIdentifier=337  MsgLength=8  SignalInfo={'LF_burst_flag','15','1','LE','unsigned','Standard','0','1','0','-Inf','Inf';'LF_burst_pressure','0','8','LE','unsigned','Standard','0','2.5','-2.5','-2.5','632.5';'LF_reserved','8','7','LE','unsigned','Standard','0','1','0','-Inf','Inf';'LR_burst_flag','31','1','LE','unsigned','Standard','0','1','0','-Inf','Inf';'LR_burst_pressure','16','8','LE','unsigned','Standard','0','2.5','-2.5','-2.5','632.5';'LR_reserved','24','7','LE','unsigned','Standard','0','1','0','-Inf','Inf';'RF_burst_flag','63','1','LE','unsigned','Standard','0','1','0','-Inf','Inf';'RF_burst_pressure','48','8','LE','unsigned','Standard','0','2.5','-2.5','-2.5','632.5';'RF_reserved','56','7','LE','unsigned','Standard','0','1','0','-Inf','Inf';'RR_burst_flag','47','1','LE','unsigned','Standard','0','1','0','-Inf','Inf';'RR_burst_pressure','32','8','LE','unsigned','Standard','0','2.5','-2.5','-2.5','632.5';'RR_reserved','40','7','LE','unsigned','Standard','0','1','0','-Inf','Inf'}  IDPort=off  TimestampPort=off  ErrorPort=off  RemotePort=off  LengthPort=off  StatusPort=off  ApplyMinMax=off
      settings: SourceProductBaseCode=ME,VN  DataFormat=CANdb specified signals
  TPMS_TireBurst*1 : Outport
  wires:
  In1/1 -> TPMS_TireBurst/1
  Bus Creator/1 -> TPMS_TireBurst*1/1  "TPMS_TireBurst"
  TPMS_TireBurst/1 -> Bus Creator/1  "LF_burst_flag"
  TPMS_TireBurst/2 -> Bus Creator/2  "LF_burst_pressure"
  TPMS_TireBurst/4 -> Bus Creator/3  "LR_burst_flag"
  TPMS_TireBurst/5 -> Bus Creator/4  "LR_burst_pressure"
  TPMS_TireBurst/11 -> Bus Creator/8  "RR_burst_pressure"
  TPMS_TireBurst/10 -> Bus Creator/7  "RR_burst_flag"
  TPMS_TireBurst/8 -> Bus Creator/6  "RF_burst_pressure"
  TPMS_TireBurst/7 -> Bus Creator/5  "RF_burst_flag"
